simulink model "Wii_Falcon"  (Simulink 7.0)
settings: Solver=ode1  StartTime=0.0  StopTime=inf  FixedStep=0.001  RelTol=1e-3
undefined symbols (not defined in the file or in its folder): X, Y, Z
libraries: quarc_library x1
settings Model: Creator=colinlea  LastModifiedBy=colinlea  ExtModeTrigDuration=10000
settings SolverCC: PositivePriorityOrder=on
settings RTWCC: SystemTargetFile=quarc_windows.tlc  TemplateMakefile=quarc_default_tmf  Description=QuaRC Win32 Target  ProcessScript=quarc_windows_make_rtw_hook
settings STFCustomTargetCC: TargetPreCompLibLocation=C:\DOCUME~1\ALLUSE~1\APPLIC~1\QuaRC\lib\2007b\windows\release  GenFloatMathFcnCalls=ANSI_C  SystemTargetFile=quarc_windows.tlc
settings GRTTargetCC: TargetPreCompLibLocation=C:\DOCUME~1\ALLUSE~1\APPLIC~1\QuaRC\lib\2007b\windows\release  CompOptLevelCompliant=off  MatFileLogging=off  ExtMode=on  ExtModeMexFile=quarc_comm

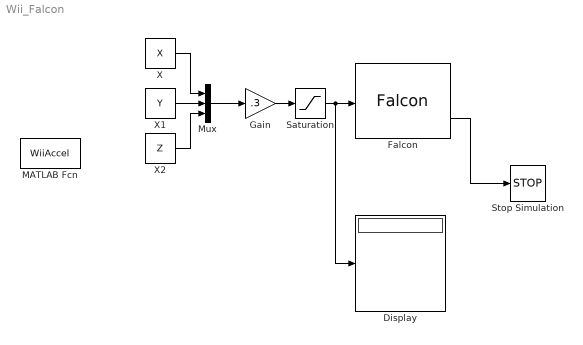
== system Wii_Falcon ==
  Display : Display
  Falcon : quarc_library/Devices/Third-Party/Novint/Falcon  sample_time=qc_get_step_size  show_calibrate=off
  Gain : Gain  Gain=.3  ParameterDataType=sfix(16)  ParameterScaling=2^0  OutDataType=sfix(16)  OutScaling=2^0
  MATLAB Fcn : MATLABFcn  MATLABFcn=WiiAccel
  Mux : Mux  Inputs=3
  Saturation : Saturate  UpperLimit=4  LowerLimit=-4  OutDataType=sfix(16)  OutScaling=2^0
  Stop Simulation : Stop
  X : Constant  Value=X  OutDataType=sfix(16)  OutScaling=2^0
  X1 : Constant  Value=Y  OutDataType=sfix(16)  OutScaling=2^0
  X2 : Constant  Value=Z  OutDataType=sfix(16)  OutScaling=2^0
  wires:
  Gain/1 -> Saturation/1
  Falcon/2 -> Stop Simulation/1
  X/1 -> Mux/1
  X1/1 -> Mux/2
  X2/1 -> Mux/3
  Mux/1 -> Gain/1
  Saturation/1 -> Falcon/1, Display/1
